simulink library "controllerForDoublePendulum"  (R2017b)
settings: Solver=VariableStepAuto  StartTime=0.0  StopTime=10.0  RelTol=1e-3
undefined symbols (not defined in the file): initFeedback
settings Model: Creator=muralikarnam  LastModifiedBy=muralikarnam

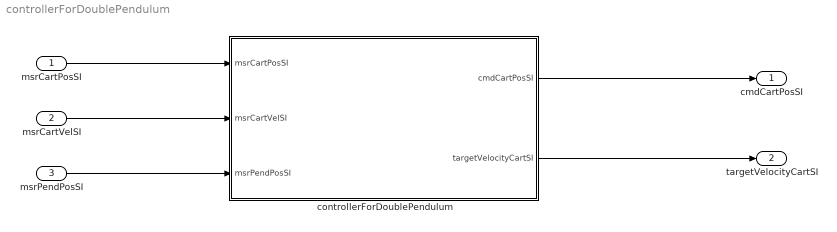
== system controllerForDoublePendulum ==
  msrCartPosSI : Inport  OutDataTypeStr=double  PortDimensions=2
  msrCartVelSI : Inport  Port=2  OutDataTypeStr=double  PortDimensions=2
  msrPendPosSI : Inport  Port=3  OutDataTypeStr=double  PortDimensions=2
  controllerForDoublePendulum : Subsystem
  cmdCartPosSI : Outport  OutDataTypeStr=double  PortDimensions=2
  targetVelocityCartSI : Outport  Port=2  OutDataTypeStr=double  PortDimensions=2
  wires:
  msrCartPosSI/1 -> controllerForDoublePendulum/1(msrCartPosSI)
  msrCartVelSI/1 -> controllerForDoublePendulum/2(msrCartVelSI)
  msrPendPosSI/1 -> controllerForDoublePendulum/3(msrPendPosSI)
  controllerForDoublePendulum/1(cmdCartPosSI) -> cmdCartPosSI/1
  controllerForDoublePendulum/2(targetVelocityCartSI) -> targetVelocityCartSI/1

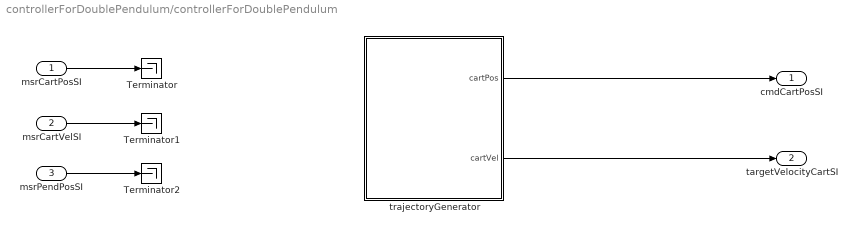
== system controllerForDoublePendulum/controllerForDoublePendulum ==
  msrCartPosSI : Inport  OutDataTypeStr=double  PortDimensions=2
  msrCartVelSI : Inport  Port=2  OutDataTypeStr=double  PortDimensions=2
  msrPendPosSI : Inport  Port=3  OutDataTypeStr=double  PortDimensions=2
  Terminator : Terminator
  Terminator1 : Terminator
  Terminator2 : Terminator
  trajectoryGenerator : Subsystem
  cmdCartPosSI : Outport  OutDataTypeStr=double  PortDimensions=2
  targetVelocityCartSI : Outport  Port=2  OutDataTypeStr=double  PortDimensions=2
  wires:
  msrPendPosSI/1 -> Terminator2/1
  trajectoryGenerator/2(cartVel) -> targetVelocityCartSI/1
  msrCartVelSI/1 -> Terminator1/1
  msrCartPosSI/1 -> Terminator/1
  trajectoryGenerator/1(cartPos) -> cmdCartPosSI/1

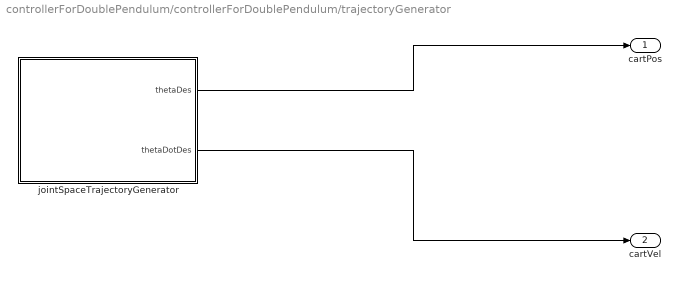
== system controllerForDoublePendulum/controllerForDoublePendulum/trajectoryGenerator ==
  jointSpaceTrajectoryGenerator : Subsystem
  cartPos : Outport
  cartVel : Outport  Port=2
  wires:
  jointSpaceTrajectoryGenerator/1(thetaDes) -> cartPos/1
  jointSpaceTrajectoryGenerator/2(thetaDotDes) -> cartVel/1

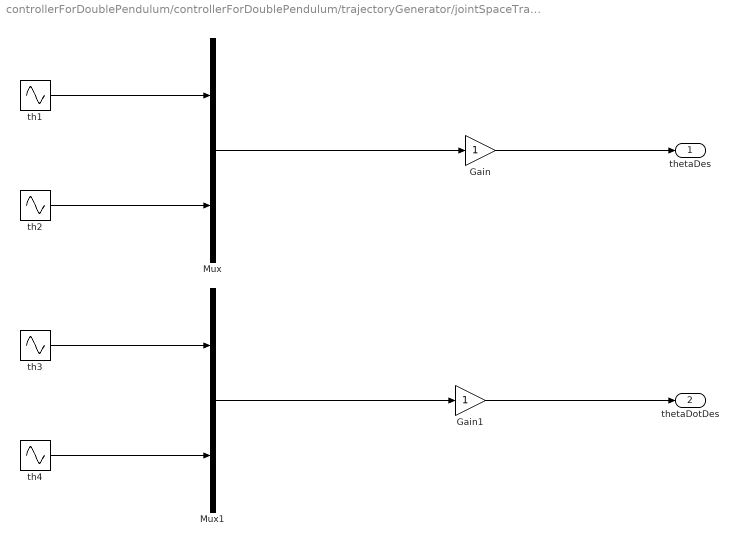
== system controllerForDoublePendulum/controllerForDoublePendulum/trajectoryGenerator/jointSpaceTrajectoryGenerator ==
  Gain : Gain
  Gain1 : Gain
  Mux : Mux  Inputs=2
  Mux1 : Mux  Inputs=2
  th1 : Sin  Amplitude=0.1  Bias=initFeedback.cartPos(1)  Frequency=10  SampleTime=0
  th2 : Sin  Amplitude=0.1  Bias=initFeedback.cartPos(2)  Frequency=5  SampleTime=0
  th3 : Sin  Frequency=10  SampleTime=0
  th4 : Sin  Amplitude=0.5  Frequency=5  SampleTime=0
  thetaDes : Outport
  thetaDotDes : Outport  Port=2
  wires:
  Mux/1 -> Gain/1
  th2/1 -> Mux/2
  th1/1 -> Mux/1
  Mux1/1 -> Gain1/1
  th3/1 -> Mux1/1
  th4/1 -> Mux1/2
  Gain/1 -> thetaDes/1
  Gain1/1 -> thetaDotDes/1
